simulink subsystem "c_rating"  (R2024b)
settings: Solver=VariableStepAuto  StartTime=0.0  StopTime=10.0  RelTol=1e-3
model mask{i_worst=0, cap_b=0}
  mask prompts: i_worst "Worst case current (A)"; cap_b "Cell capacity (Ah)"
settings Model: Creator=Mohammed Hany  LastModifiedBy=Mohammed Hany

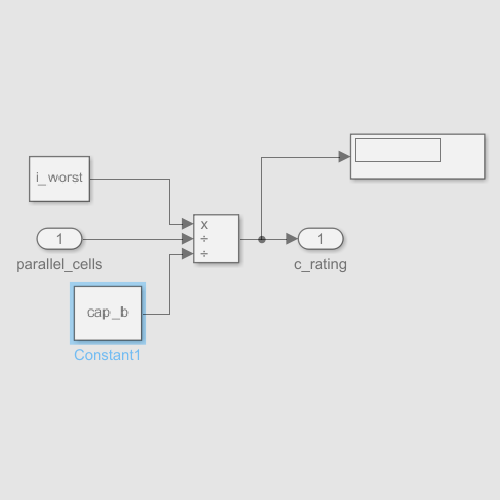
[thumbnail: Simulink's stored preview of the top-level diagram]
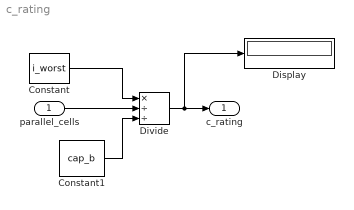
== system c_rating ==
  parallel_cells : Inport
  Constant : Constant  Value=i_worst
  Constant1 : Constant  Value=cap_b
  Display : Display
  Divide : Product  Inputs=*//
  c_rating : Outport
  wires:
  Divide/1 -> c_rating/1, Display/1
  parallel_cells/1 -> Divide/2
  Constant/1 -> Divide/1
  Constant1/1 -> Divide/3
